simulink model "Q2"  (R2025a)
settings: Solver=VariableStepAuto  StartTime=0.0  StopTime=15  RelTol=1e-3
settings Model: Creator=64892  LastModifiedBy=64892

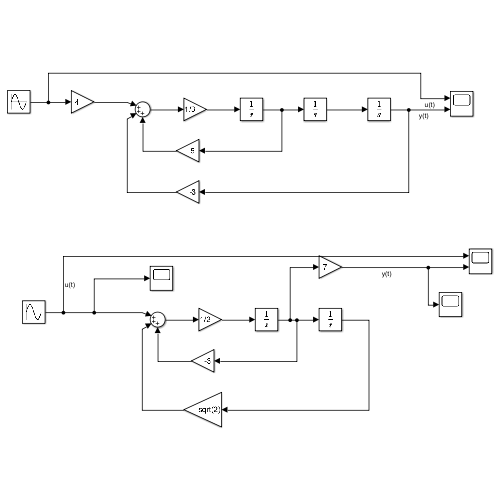
[thumbnail: Simulink's stored preview of the top-level diagram]
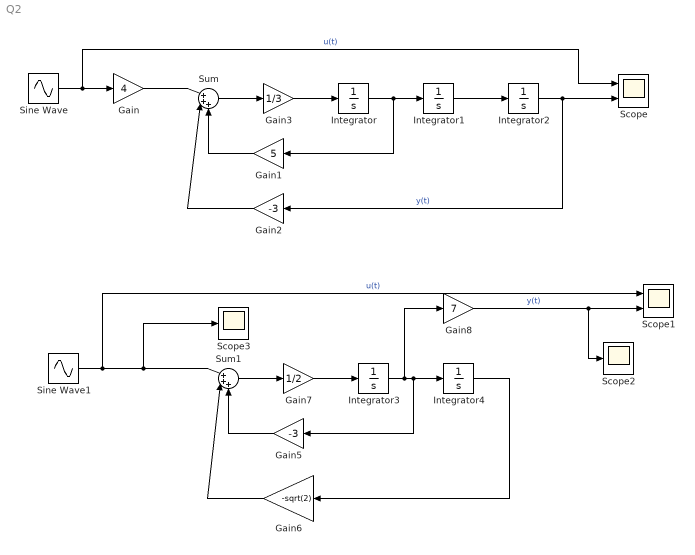
== system Q2 ==
  Gain : Gain  Gain=4
  Gain1 : Gain  Gain=5
  Gain2 : Gain  Gain=-3
  Gain3 : Gain  Gain=1/3
  Gain5 : Gain  Gain=-3
  Gain6 : Gain  Gain=-sqrt(2)
  Gain7 : Gain  Gain=1/2
  Gain8 : Gain  Gain=7
  Integrator{,1..4} (5 alike) : Integrator
  Scope : Scope  NumInputPorts=2
      settings: ActiveDisplayYMinimum=-34973.474110531424  ActiveDisplayYMaximum=7678.7382214928784
  Scope1 : Scope  NumInputPorts=2
      settings: ActiveDisplayYMinimum=-26.798266941516349  ActiveDisplayYMaximum=18.352257346754648
  Scope2 : Scope
      settings: ActiveDisplayYMinimum=-1  ActiveDisplayYMaximum=1  DataLoggingVariableName=ScopeData2
  Scope3 : Scope
      settings: ActiveDisplayYMinimum=-1  ActiveDisplayYMaximum=1  DataLoggingVariableName=ScopeData3
  Sine Wave : Sin  SampleTime=0
  Sine Wave1 : Sin  SampleTime=0
  Sum : Sum  Inputs=|+++
  Sum1 : Sum  Inputs=|+++
  wires:
  Gain/1 -> Sum/1
  Sum/1 -> Gain3/1
  Gain1/1 -> Sum/3
  Gain2/1 -> Sum/2
  Gain3/1 -> Integrator/1
  Integrator/1 -> Gain1/1, Integrator1/1
  Integrator1/1 -> Integrator2/1
  Integrator2/1 -> Scope/2, Gain2/1  "y(t)"
  Sine Wave/1 -> Scope/1, Gain/1  "u(t)"
  Integrator4/1 -> Gain6/1
  Sum1/1 -> Gain7/1
  Gain7/1 -> Integrator3/1
  Gain5/1 -> Sum1/3
  Sine Wave1/1 -> Scope1/1, Sum1/1, Scope3/1  "u(t)"
  Integrator3/1 -> Gain8/1, Gain5/1, Integrator4/1
  Gain6/1 -> Sum1/2
  Gain8/1 -> Scope2/1, Scope1/2  "y(t)"
